simulink model "ForwardKinematic_YuMi"  (R2024a)
(part 15 of 23)

cos(q2L)*((4872700232219253*cos(q1L))/9007199254740992 + (6283307137322267*sin(q1L))/9007199254740992) - (7514214926474921*sin(q2L)*((6283307137322267*cos(q1L))/9007199254740992 - (4872700232219253*sin(q1L))/9007199254740992))/36893488147419103232) + (7514214926474921*sin(q3L)*((7514214926474921*cos(q2L)*((6283307137322267*cos(q1L))/9007199254740992 - (4872700232219253*sin(q1L))/9007199254740992))/36893488147419103232 - (76229820211215127867025072518845*cos(q2L))/162259276829213363391578010288128 + sin(q2L)*((4872700232219253*cos(q1L))/9007199254740992 + (6283307137322267*sin(q1L))/9007199254740992)))/36893488147419103232) + ((234819211581865*cos(q4L))/1152921504606846976 + (9007199067919185*sin(q4L))/9007199254740992)*((425266980168672787164801917791314326747055225795*cos(q1L))/2993155353253689176481146537402947624255349848014848 + (686617165554103949950999710565799465200849541325*cos(q2L))/1461501637330902918203684832716283019655932542976 - (329794241748012540206902858004467560228111939405*sin(q1L))/2993155353253689176481146537402947624255349848014848 - (67682029681889335677290557259385*cos(q2L)*((6283307137322267*cos(q1L))/9007199254740992 - (4872700232219253*sin(q1L))/9007199254740992))/332306998946228968225951765070086144 - (9007199067919185*sin(q2L)*((4872700232219253*cos(q1L))/9007199254740992 + (6283307137322267*sin(q1L))/9007199254740992))/9007199254740992 + 477861849958017465213997854626476001002268408317/24519928653854221733733552434404946937899825954937634816) + (7514214926474921*cos(q4L)*((9007199067919185*cos(q3L)*((56594998190739085871744456992395*cos(q1L))/81129638414606681695789005144064 - (43889380989894851923989405068805*sin(q1L))/81129638414606681695789005144064 + 63594381400292563045725890951477/664613997892457936451903530140172288))/9007199254740992 + (7514214926474921*cos(q3L)*((7514214926474921*cos(q2L)*((6283307137322267*cos(q1L))/9007199254740992 - (4872700232219253*sin(q1L))/9007199254740992))/36893488147419103232 - (76229820211215127867025072518845*cos(q2L))/162259276829213363391578010288128 + sin(q2L)*((4872700232219253*cos(q1L))/9007199254740992 + (6283307137322267*sin(q1L))/9007199254740992)))/36893488147419103232 - sin(q3L)*((76229820211215127867025072518845*sin(q2L))/162259276829213363391578010288128 + cos(q2L)*((4872700232219253*cos(q1L))/9007199254740992 + (6283307137322267*sin(q1L))/9007199254740992) - (7514214926474921*sin(q2L)*((6283307137322267*cos(q1L))/9007199254740992 - (4872700232219253*sin(q1L))/9007199254740992))/36893488147419103232)))/36893488147419103232))/36893488147419103232 + cos(q5L)*(((7514214926474921*cos(q4L))/36893488147419103232 + (4503599440548691*sin(q4L))/4503599627370496)*((9007199067919185*sin(q3L)*((56594998190739085871744456992395*cos(q1L))/81129638414606681695789005144064 - (43889380989894851923989405068805*sin(q1L))/81129638414606681695789005144064 + 63594381400292563045725890951477/664613997892457936451903530140172288))/9007199254740992 + cos(q3L)*((76229820211215127867025072518845*sin(q2L))/162259276829213363391578010288128 + cos(q2L)*((4872700232219253*cos(q1L))/9007199254740992 + (6283307137322267*sin(q1L))/9007199254740992) - (7514214926474921*sin(q2L)*((6283307137322267*cos(q1L))/9007199254740992 - (4872700232219253*sin(q1L))/9007199254740992))/36893488147419103232) + (7514214926474921*sin(q3L)*((7514214926474921*cos(q2L)*((6283307137322267*cos(q1L))/9007199254740992 - (4872700232219253*sin(q1L))/9007199254740992))/36893488147419103232 - (76229820211215127867025072518845*cos(q2L))/162259276829213363391578010288128 + sin(q2L)*((4872700232219253*cos(q1L))/9007199254740992 + (6283307137322267*sin(q1L))/9007199254740992)))/36893488147419103232) - ((9007199067919185*cos(q4L))/9007199254740992 - (234819211581865*sin(q4L))/1152921504606846976)*((425266980168672787164801917791314326747055225795*cos(q1L))/2993155353253689176481146537402947624255349848014848 + (686617165554103949950999710565799465200849541325*cos(q2L))/1461501637330902918203684832716283019655932542976 - (329794241748012540206902858004467560228111939405*sin(q1L))/2993155353253689176481146537402947624255349848014848 - (67682029681889335677290557259385*cos(q2L)*((6283307137322267*cos(q1L))/9007199254740992 - (4872700232219253*sin(q1L))/9007199254740992))/332306998946228968225951765070086144 - (9007199067919185*sin(q2L)*((4872700232219253*cos(q1L))/9007199254740992 + (6283307137322267*sin(q1L))/9007199254740992))/9007199254740992 + 477861849958017465213997854626476001002268408317/24519928653854221733733552434404946937899825954937634816) + (7514214926474921*sin(q4L)*((9007199067919185*cos(q3L)*((56594998190739085871744456992395*cos(q1L))/81129638414606681695789005144064 - (43889380989894851923989405068805*sin(q1L))/81129638414606681695789005144064 + 63594381400292563045725890951477/664613997892457936451903530140172288))/9007199254740992 + (7514214926474921*cos(q3L)*((7514214926474921*cos(q2L)*((6283307137322267*cos(q1L))/9007199254740992 - (4872700232219253*sin(q1L))/9007199254740992))/36893488147419103232 - (76229820211215127867025072518845*cos(q2L))/162259276829213363391578010288128 + sin(q2L)*((4872700232219253*cos(q1L))/9007199254740992 + (6283307137322267*sin(q1L))/9007199254740992)))/36893488147419103232 - sin(q3L)*((76229820211215127867025072518845*sin(q2L))/162259276829213363391578010288128 + cos(q2L)*((4872700232219253*cos(q1L))/9007199254740992 + (6283307137322267*sin(q1L))/9007199254740992) - (7514214926474921*sin(q2L)*((6283307137322267*cos(q1L))/9007199254740992 - (4872700232219253*sin(q1L))/9007199254740992))/36893488147419103232)))/36893488147419103232)))/9007199254740992000 + (2436553109258773196144549622003023*sin(q6L)*((7514214926474921*cos(q5L)*(((4503599440548691*cos(q4L))/4503599627370496 - (7514214926474921*sin(q4L))/36893488147419103232)*((9007199067919185*sin(q3L)*((56594998190739085871744456992395*cos(q1L))/81129638414606681695789005144064 - (43889380989894851923989405068805*sin(q1L))/81129638414606681695789005144064 + 63594381400292563045725890951477/664613997892457936451903530140172288))/9007199254740992 + cos(q3L)*((76229820211215127867025072518845*sin(q2L))/162259276829213363391578010288128 + cos(q2L)*((4872700232219253*cos(q1L))/9007199254740992 + (6283307137322267*sin(q1L))/9007199254740992) - (7514214926474921*sin(q2L)*((6283307137322267*cos(q1L))/9007199254740992 - (4872700232219253*sin(q1L))/9007199254740992))/36893488147419103232) + (7514214926474921*sin(q3L)*((7514214926474921*cos(q2L)*((6283307137322267*cos(q1L))/9007199254740992 - (4872700232219253*sin(q1L))/9007199254740992))/36893488147419103232 - (76229820211215127867025072518845*cos(q2L))/162259276829213363391578010288128 + sin(q2L)*((4872700232219253*cos(q1L))/9007199254740992 + (6283307137322267*sin(q1L))/9007199254740992)))/36893488147419103232) + ((234819211581865*cos(q4L))/1152921504606846976 + (9007199067919185*sin(q4L))/9007199254740992)*((425266980168672787164801917791314326747055225795*cos(q1L))/2993155353253689176481146537402947624255349848014848 + (686617165554103949950999710565799465200849541325*cos(q2L))/1461501637330902918203684832716283019655932542976 - (329794241748012540206902858004467560228111939405*sin(q1L))/2993155353253689176481146537402947624255349848014848 - (67682029681889335677290557259385*cos(q2L)*((6283307137322267*cos(q1L))/9007199254740992 - (4872700232219253*sin(q1L))/9007199254740992))/332306998946228968225951765070086144 - (9007199067919185*sin(q2L)*((4872700232219253*cos(q1L))/9007199254740992 + (6283307137322267*sin(q1L))/9007199254740992))/9007199254740992 + 477861849958017465213997854626476001002268408317/24519928653854221733733552434404946937899825954937634816) + (7514214926474921*cos(q4L)*((9007199067919185*cos(q3L)*((56594998190739085871744456992395*cos(q1L))/81129638414606681695789005144064 - (43889380989894851923989405068805*sin(q1L))/81129638414606681695789005144064 + 63594381400292563045725890951477/664613997892457936451903530140172288))/9007199254740992 + (7514214926474921*cos(q3L)*((7514214926474921*cos(q2L)*((6283307137322267*cos(q1L))/9007199254740992 - (4872700232219253*sin(q1L))/9007199254740992))/36893488147419103232 - (76229820211215127867025072518845*cos(q2L))/162259276829213363391578010288128 + sin(q2L)*((4872700232219253*cos(q1L))/9007199254740992 + (6283307137322267*sin(q1L))/9007199254740992)))/36893488147419103232 - sin(q3L)*((76229820211215127867025072518845*sin(q2L))/162259276829213363391578010288128 + cos(q2L)*((4872700232219253*cos(q1L))/9007199254740992 + (6283307137322267*sin(q1L))/9007199254740992) - (7514214926474921*sin(q2L)*((6283307137322267*cos(q1L))/9007199254740992 - (4872700232219253*sin(q1L))/9007199254740992))/36893488147419103232)))/36893488147419103232))/36893488147419103232 - (9007199067919185*cos(q5L)*((666467732349846997487583938718911583194406904318712922873589125*cos(q1L))/113078212145816597093331040047546785012958969400039613319782796882727665664 + (1076049180065244948668759145796765391250102872519935285209856875*cos(q2L))/55213970774324510299478046898216203619608871777363092441300193790394368 - (516845254133432670685844229576986303733782399690601453662320875*sin(q1L))/113078212145816597093331040047546785012958969400039613319782796882727665664 - (81129635049124235038645691064225*cos(q3L)*((56594998190739085871744456992395*cos(q1L))/81129638414606681695789005144064 - (43889380989894851923989405068805*sin(q1L))/81129638414606681695789005144064 + 63594381400292563045725890951477/664613997892457936451903530140172288))/81129638414606681695789005144064 + (2115063383689692319117831580025*sin(q3L)*((56594998190739085871744456992395*cos(q1L))/81129638414606681695789005144064 - (43889380989894851923989405068805*sin(q1L))/81129638414606681695789005144064 + 63594381400292563045725890951477/664613997892457936451903530140172288))/10384593717069655257060992658440192 - (67682029681889335677290557259385*cos(q3L)*((7514214926474921*cos(q2L)*((6283307137322267*cos(q1L))/9007199254740992 - (4872700232219253*sin(q1L))/9007199254740992))/36893488147419103232 - (76229820211215127867025072518845*cos(q2L))/162259276829213363391578010288128 + sin(q2L)*((4872700232219253*cos(q1L))/9007199254740992 + (6283307137322267*sin(q1L))/9007199254740992)))/332306998946228968225951765070086144 + (234819211581865*cos(q3L)*((76229820211215127867025072518845*sin(q2L))/162259276829213363391578010288128 + cos(q2L)*((4872700232219253*cos(q1L))/9007199254740992 + (6283307137322267*sin(q1L))/9007199254740992) - (7514214926474921*sin(q2L)*((6283307137322267*cos(q1L))/9007199254740992 - (4872700232219253*sin(q1L))/9007199254740992))/36893488147419103232))/1152921504606846976 + (1764482024691522628700660907665*sin(q3L)*((7514214926474921*cos(q2L)*((6283307137322267*cos(q1L))/9007199254740992 - (4872700232219253*sin(q1L))/9007199254740992))/36893488147419103232 - (76229820211215127867025072518845*cos(q2L))/162259276829213363391578010288128 + sin(q2L)*((4872700232219253*cos(q1L))/9007199254740992 + (6283307137322267*sin(q1L))/9007199254740992)))/42535295865117307932921825928971026432 + (9007199067919185*sin(q3L)*((76229820211215127867025072518845*sin(q2L))/162259276829213363391578010288128 + cos(q2L)*((4872700232219253*cos(q1L))/9007199254740992 + (6283307137322267*sin(q1L))/9007199254740992) - (7514214926474921*sin(q2L)*((6283307137322267*cos(q1L))/9007199254740992 - (4872700232219253*sin(q1L))/9007199254740992))/36893488147419103232))/9007199254740992 - (106069577339469832923929692356850887620017617375*cos(q2L)*((6283307137322267*cos(q1L))/9007199254740992 - (4872700232219253*sin(q1L))/9007199254740992))/12554203470773361527671578846415332832204710888928069025792 - (14115856197532180673579726082375*sin(q2L)*((4872700232219253*cos(q1L))/9007199254740992 + (6283307137322267*sin(q1L))/9007199254740992))/340282366920938463463374607431768211456 + 748893091562634003789577347105888574211761174637088840996300475/926336713898529563388567880069503262826159877325124512315660672063305037119488))/9007199254740992 + sin(q5L)*(((7514214926474921*cos(q4L))/36893488147419103232 + (4503599440548691*sin(q4L))/4503599627370496)*((9007199067919185*sin(q3L)*((56594998190739085871744456992395*cos(q1L))/81129638414606681695789005144064 - (43889380989894851923989405068805*sin(q1L))/81129638414606681695789005144064 + 63594381400292563045725890951477/664613997892457936451903530140172288))/9007199254740992 + cos(q3L)*((76229820211215127867025072518845*sin(q2L))/162259276829213363391578010288128 + cos(q2L)*((4872700232219253*cos(q1L))/9007199254740992 + (6283307137322267*sin(q1L))/9007199254740992) - (7514214926474921*sin(q2L)*((6283307137322267*cos(q1L))/9007199254740992 - (4872700232219253*sin(q1L))/9007199254740992))/36893488147419103232) + (7514214926474921*sin(q3L)*((7514214926474921*cos(q2L)*((6283307137322267*cos(q1L))/9007199254740992 - (4872700232219253*sin(q1L))/9007199254740992))/36893488147419103232 - (76229820211215127867025072518845*cos(q2L))/162259276829213363391578010288128 + sin(q2L)*((4872700232219253*cos(q1L))/9007199254740992 + (6283307137322267*sin(q1L))/9007199254740992)))/36893488147419103232) - ((9007199067919185*cos(q4L))/9007199254740992 - (234819211581865*sin(q4L))/1152921504606846976)*((425266980168672787164801917791314326747055225795*cos(q1L))/2993155353253689176481146537402947624255349848014848 + (686617165554103949950999710565799465200849541325*cos(q2L))/1461501637330902918203684832716283019655932542976 - (329794241748012540206902858004467560228111939405*sin(q1L))/2993155353253689176481146537402947624255349848014848 - (67682029681889335677290557259385*cos(q2L)*((6283307137322267*cos(q1L))/9007199254740992 - (4872700232219253*sin(q1L))/9007199254740992))/332306998946228968225951765070086144 - (9007199067919185*sin(q2L)*((4872700232219253*cos(q1L))/9007199254740992 + (6283307137322267*sin(q1L))/9007199254740992))/9007199254740992 + 477861849958017465213997854626476001002268408317/24519928653854221733733552434404946937899825954937634816) + (7514214926474921*sin(q4L)*((9007199067919185*cos(q3L)*((56594998190739085871744456992395*cos(q1L))/81129638414606681695789005144064 - (43889380989894851923989405068805*sin(q1L))/81129638414606681695789005144064 + 63594381400292563045725890951477/664613997892457936451903530140172288))/9007199254740992 + (7514214926474921*cos(q3L)*((7514214926474921*cos(q2L)*((6283307137322267*cos(q1L))/9007199254740992 - (4872700232219253*sin(q1L))/9007199254740992))/36893488147419103232 - (76229820211215127867025072518845*cos(q2L))/162259276829213363391578010288128 + sin(q2L)*((4872700232219253*cos(q1L))/9007199254740992 + (6283307137322267*sin(q1L))/9007199254740992)))/36893488147419103232 - sin(q3L)*((76229820211215127867025072518845*sin(q2L))/162259276829213363391578010288128 + cos(q2L)*((4872700232219253*cos(q1L))/9007199254740992 + (6283307137322267*sin(q1L))/9007199254740992) - (7514214926474921*sin(q2L)*((6283307137322267*cos(q1L))/9007199254740992 - (4872700232219253*sin(q1L))/9007199254740992))/36893488147419103232)))/36893488147419103232)))/332306998946228968225951765070086144000 + (27*sin(q6L)*((9007199067919185*sin(q5L)*((666467732349846997487583938718911583194406904318712922873589125*cos(q1L))/113078212145816597093331040047546785012958969400039613319782796882727665664 + (1076049180065244948668759145796765391250102872519935285209856875*cos(q2L))/55213970774324510299478046898216203619608871777363092441300193790394368 - (516845254133432670685844229576986303733782399690601453662320875*sin(q1L))/113078212145816597093331040047546785012958969400039613319782796882727665664 - (81129635049124235038645691064225*cos(q3L)*((56594998190739085871744456992395*cos(q1L))/81129638414606681695789005144064 - (43889380989894851923989405068805*sin(q1L))/81129638414606681695789005144064 + 63594381400292563045725890951477/664613997892457936451903530140172288))/81129638414606681695789005144064 + (2115063383689692319117831580025*sin(q3L)*((56594998190739085871744456992395*cos(q1L))/81129638414606681695789005144064 - (43889380989894851923989405068805*sin(q1L))/81129638414606681695789005144064 + 63594381400292563045725890951477/664613997892457936451903530140172288))/10384593717069655257060992658440192 - (67682029681889335677290557259385*cos(q3L)*((7514214926474921*cos(q2L)*((6283307137322267*cos(q1L))/9007199254740992 - (4872700232219253*sin(q1L))/9007199254740992))/36893488147419103232 - (76229820211215127867025072518845*cos(q2L))/162259276829213363391578010288128 + sin(q2L)*((4872700232219253*cos(q1L))/9007199254740992 + (6283307137322267*sin(q1L))/9007199254740992)))/332306998946228968225951765070086144 + (234819211581865*cos(q3L)*((76229820211215127867025072518845*sin(q2L))/162259276829213363391578010288128 + cos(q2L)*((4872700232219253*cos(q1L))/9007199254740992 + (6283307137322267*sin(q1L))/9007199254740992) - (7514214926474921*sin(q2L)*((6283307137322267*cos(q1L))/9007199254740992 - (4872700232219253*sin(q1L))/9007199254740992))/36893488147419103232))/1152921504606846976 + (1764482024691522628700660907665*sin(q3L)*((7514214926474921*cos(q2L)*((6283307137322267*cos(q1L))/9007199254740992 - (4872700232219253*sin(q1L))/9007199254740992))/36893488147419103232 - (76229820211215127867025072518845*cos(q2L))/162259276829213363391578010288128 + sin(q2L)*((4872700232219253*cos(q1L))/9007199254740992 + (6283307137322267*sin(q1L))/9007199254740992)))/42535295865117307932921825928971026432 + (9007199067919185*sin(q3L)*((76229820211215127867025072518845*sin(q2L))/162259276829213363391578010288128 + cos(q2L)*((4872700232219253*cos(q1L))/9007199254740992 + (6283307137322267*sin(q1L))/9007199254740992) - (7514214926474921*sin(q2L)*((6283307137322267*cos(q1L))/9007199254740992 - (4872700232219253*sin(q1L))/9007199254740992))/36893488147419103232))/9007199254740992 - (106069577339469832923929692356850887620017617375*cos(q2L)*((6283307137322267*cos(q1L))/9007199254740992 - (4872700232219253*sin(q1L))/9007199254740992))/12554203470773361527671578846415332832204710888928069025792 - (14115856197532180673579726082375*sin(q2L)*((4872700232219253*cos(q1L))/9007199254740992 + (6283307137322267*sin(q1L))/9007199254740992))/340282366920938463463374607431768211456 + 748893091562634003789577347105888574211761174637088840996300475/926336713898529563388567880069503262826159877325124512315660672063305037119488))/9007199254740992 - (7514214926474921*sin(q5L)*(((4503599440548691*cos(q4L))/4503599627370496 - (7514214926474921*sin(q4L))/36893488147419103232)*((9007199067919185*sin(q3L)*((56594998190739085871744456992395*cos(q1L))/81129638414606681695789005144064 - (43889380989894851923989405068805*sin(q1L))/81129638414606681695789005144064 + 63594381400292563045725890951477/664613997892457936451903530140172288))/9007199254740992 + cos(q3L)*((76229820211215127867025072518845*sin(q2L))/162259276829213363391578010288128 + cos(q2L)*((4872700232219253*cos(q1L))/9007199254740992 + (6283307137322267*sin(q1L))/9007199254740992) - (7514214926474921*sin(q2L)*((6283307137322267*cos(q1L))/9007199254740992 - (4872700232219253*sin(q1L))/9007199254740992))/36893488147419103232) + (7514214926474921*sin(q3L)*((7514214926474921*cos(q2L)*((6283307137322267*cos(q1L))/9007199254740992 - (4872700232219253*sin(q1L))/9007199254740992))/36893488147419103232 - (76229820211215127867025072518845*cos(q2L))/162259276829213363391578010288128 + sin(q2L)*((4872700232219253*cos(q1L))/9007199254740992 + (6283307137322267*sin(q1L))/9007199254740992)))/36893488147419103232) + ((234819211581865*cos(q4L))/1152921504606846976 + (9007199067919185*sin(q4L))/9007199254740992)*((425266980168672787164801917791314326747055225795*cos(q1L))/2993155353253689176481146537402947624255349848014848 + (686617165554103949950999710565799465200849541325*cos(q2L))/1461501637330902918203684832716283019655932542976 - (329794241748012540206902858004467560228111939405*sin(q1L))/2993155353253689176481146537402947624255349848014848 - (67682029681889335677290557259385*cos(q2L)*((6283307137322267*cos(q1L))/9007199254740992 - (4872700232219253*sin(q1L))/9007199254740992))/332306998946228968225951765070086144 - (9007199067919185*sin(q2L)*((4872700232219253*cos(q1L))/9007199254740992 + (6283307137322267*sin(q1L))/9007199254740992))/9007199254740992 + 477861849958017465213997854626476001002268408317/24519928653854221733733552434404946937899825954937634816) + (7514214926474921*cos(q4L)*((9007199067919185*cos(q3L)*((56594998190739085871744456992395*cos(q1L))/81129638414606681695789005144064 - (43889380989894851923989405068805*sin(q1L))/81129638414606681695789005144064 + 63594381400292563045725890951477/664613997892457936451903530140172288))/9007199254740992 + (7514214926474921*cos(q3L)*((7514214926474921*cos(q2L)*((6283307137322267*cos(q1L))/9007199254740992 - (4872700232219253*sin(q1L))/9007199254740992))/36893488147419103232 - (76229820211215127867025072518845*cos(q2L))/162259276829213363391578010288128 + sin(q2L)*((4872700232219253*cos(q1L))/9007199254740992 + (6283307137322267*sin(q1L))/9007199254740992)))/36893488147419103232 - sin(q3L)*((76229820211215127867025072518845*sin(q2L))/162259276829213363391578010288128 + cos(q2L)*((4872700232219253*cos(q1L))/9007199254740992 + (6283307137322267*sin(q1L))/9007199254740992) - (7514214926474921*sin(q2L)*((6283307137322267*cos(q1L))/9007199254740992 - (4872700232219253*sin(q1L))/9007199254740992))/36893488147419103232)))/36893488147419103232))/36893488147419103232 + cos(q5L)*(((7514214926474921*cos(q4L))/36893488147419103232 + (4503599440548691*sin(q4L))/4503599627370496)*((9007199067919185*sin(q3L)*((56594998190739085871744456992395*cos(q1L))/81129638414606681695789005144064 - (43889380989894851923989405068805*sin(q1L))/81129638414606681695789005144064 + 63594381400292563045725890951477/664613997892457936451903530140172288))/9007199254740992 + cos(q3L)*((76229820211215127867025072518845*sin(q2L))/162259276829213363391578010288128 + cos(q2L)*((4872700232219253*cos(q1L))/9007199254740992 + (6283307137322267*sin(q1L))/9007199254740992) - (7514214926474921*sin(q2L)*((6283307137322267*cos(q1L))/9007199254740992 - (4872700232219253*sin(q1L))/9007199254740992))/36893488147419103232) + (7514214926474921*sin(q3L)*((7514214926474921*cos(q2L)*((6283307137322267*cos(q1L))/9007199254740992 - (4872700232219253*sin(q1L))/9007199254740992))/36893488147419103232 - (76229820211215127867025072518845*cos(q2L))/162259276829213363391578010288128 + sin(q2L)*((4872700232219253*cos(q1L))/9007199254740992 + (6283307137322267*sin(q1L))/9007199254740992)))/36893488147419103232) - ((9007199067919185*cos(q4L))/9007199254740992 - (234819211581865*sin(q4L))/1152921504606846976)*((425266980168672787164801917791314326747055225795*cos(q1L))/2993155353253689176481146537402947624255349848014848 + (686617165554103949950999710565799465200849541325*cos(q2L))/1461501637330902918203684832716283019655932542976 - (329794241748012540206902858004467560228111939405*sin(q1L))/2993155353253689176481146537402947624255349848014848 - (67682029681889335677290557259385*cos(q2L)*((6283307137322267*cos(q1L))/9007199254740992 - (4872700232219253*sin(q1L))/9007199254740992))/332306998946228968225951765070086144 - (9007199067919185*sin(q2L)*((4872700232219253*cos(q1L))/9007199254740992 + (6283307137322267*sin(q1L))/9007199254740992))/9007199254740992 + 477861849958017465213997854626476001002268408317/24519928653854221733733552434404946937899825954937634816) + (7514214926474921*sin(q4L)*((9007199067919185*cos(q3L)*((56594998190739085871744456992395*cos(q1L))/81129638414606681695789005144064 - (43889380989894851923989405068805*sin(q1L))/81129638414606681695789005144064 + 63594381400292563045725890951477/664613997892457936451903530140172288))/9007199254740992 + (7514214926474921*cos(q3L)*((7514214926474921*cos(q2L)*((6283307137322267*cos(q1L))/9007199254740992 - (4872700232219253*sin(q1L))/9007199254740992))/36893488147419103232 - (76229820211215127867025072518845*cos(q2L))/162259276829213363391578010288128 + sin(q2L)*((4872700232219253*cos(q1L))/9007199254740992 + (6283307137322267*sin(q1L))/9007199254740992)))/36893488147419103232 - sin(q3L)*((76229820211215127867025072518845*sin(q2L))/162259276829213363391578010288128 + cos(q2L)*((4872700232219253*cos(q1L))/9007199254740992 + (6283307137322267*sin(q1L))/9007199254740992) - (7514214926474921*sin(q2L)*((6283307137322267*cos(q1L))/9007199254740992 - (4872700232219253*sin(q1L))/9007199254740992))/36893488147419103232)))/36893488147419103232)))/1000, 0];
